simulink model "ocex"  (Simulink 8.5)
settings: Solver=ode45  SolverMode=SingleTasking  StartTime=0.0  StopTime=0.1  RelTol=1e-3  AbsTol=1e-6
libraries: elements x2
settings Model: Creator=PC  LastModifiedBy=PC
settings DataIOCC: LimitDataPoints=off
settings OptimizationCC: BlockReduction=off  BooleanDataType=off  ExpressionDepthLimit=128
settings DebuggingCC: SaveWithParameterizedLinksMsg=none  SignalResolutionControl=TryResolveAllWithWarning  MultiTaskDSMMsg=warning  MultiTaskCondExecSysMsg=none  FcnCallInpInsideContextMsg=EnableAllAsError  StateNameClashWarn=none  StrictBusMsg=None
settings HardwareCC: TargetUnknown=on

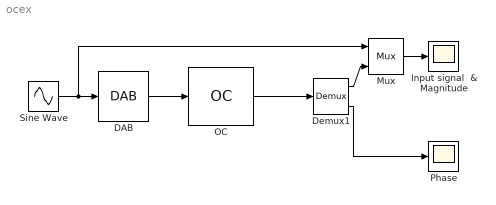
== system ocex ==
  DAB : elements/DAB  filter=on  approx=Butterworth  order=2  numerator=[]  denominator=[]  freq=180  resdis=off  vertres=8  xmax=1  winsize=40  G=1.0  fs=60*40
  Demux1 : Demux  Outputs=2
  Input signal  & Magnitude : Scope
      settings: TickLabels=on  TimeRange=0.1
  Mux : Mux  Inputs=2
  OC : elements/OC  tfilt=Walsh  rfilt=[ ]  ifilt=[ ]  tlen=half  N1=40
  Phase : Scope
      settings: TickLabels=on  TimeRange=0.1
  Sine Wave : Sin  Frequency=2*pi*60  SampleTime=0
  wires:
  Sine Wave/1 -> DAB/1, Mux/1
  DAB/1 -> OC/1
  Demux1/1 -> Mux/2
  OC/1 -> Demux1/1
  Mux/1 -> Input signal  & Magnitude/1
  Demux1/2 -> Phase/1
